simulink model "Approach_Model"  (R2017a)
settings: Solver=VariableStepAuto  StartTime=0.0  StopTime=100  RelTol=1e-3
libraries: cstblocks x1
settings Model: Creator=user  LastModifiedBy=user

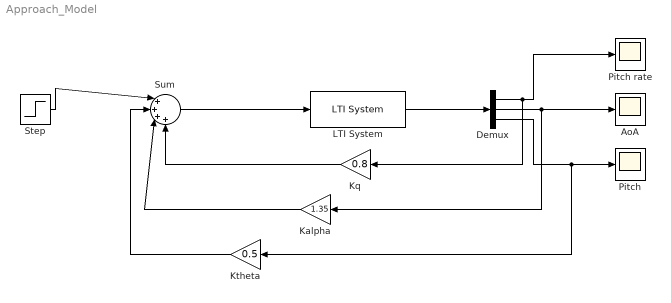
== system Approach_Model ==
  AoA : Scope
  Demux : Demux  Outputs=3
  Kalpha : Gain  Gain=1.35
  Kq : Gain  Gain=0.8
  Ktheta : Gain  Gain=0.5
  LTI System : cstblocks/LTI System  sys=Sys1  IC=[]
  Pitch : Scope
  "Pitch rate " : Scope
  Step : Step  Time=0  SampleTime=0
  Sum : Sum  Inputs=|++++
  wires:
  LTI System/1 -> Demux/1
  Demux/1 -> Kq/1, "Pitch rate "/1
  Demux/2 -> Kalpha/1, AoA/1
  Demux/3 -> Ktheta/1, Pitch/1
  Step/1 -> Sum/1
  Kq/1 -> Sum/4
  Kalpha/1 -> Sum/3
  Ktheta/1 -> Sum/2
  Sum/1 -> LTI System/1
